simulink model "set_point"  (R2023b)
settings: Solver=VariableStepAuto  StartTime=0.0  StopTime=10.0  RelTol=1e-3
values from neighbouring files (symbols this model uses):
  r = 120.0    (= 120)    [controlador_foc_simulink.m]    (also in parametros_planta.m; params_subsistema_mecanico.m; sistema_completo_en_codigo.m)
settings Model: Creator=Pc  LastModifiedBy=Pc

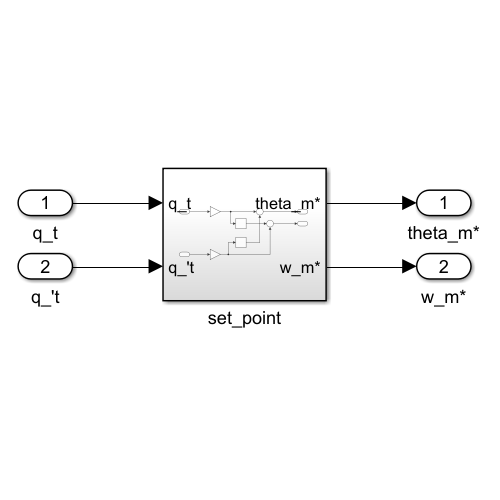
[thumbnail: Simulink's stored preview of the top-level diagram]
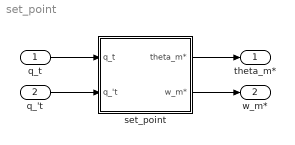
== system set_point ==
  q_t : Inport
  q_'t : Inport  Port=2
  set_point : Subsystem
  theta_m* : Outport
  w_m* : Outport  Port=2
  wires:
  q_t/1 -> set_point/1(q_t)
  q_'t/1 -> set_point/2(q_'t)
  set_point/1(theta_m*) -> theta_m*/1
  set_point/2(w_m*) -> w_m*/1

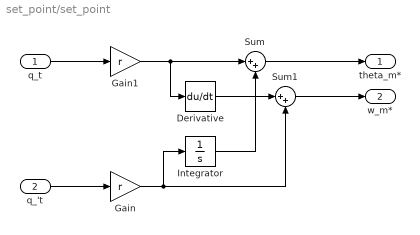
== system set_point/set_point ==
  q_t : Inport
  q_'t : Inport  Port=2
  Derivative : Derivative
  Gain : Gain  Gain=r
  Gain1 : Gain  Gain=r
  Integrator : Integrator
  Sum : Sum  Inputs=|++
  Sum1 : Sum  Inputs=|++
  theta_m* : Outport
  w_m* : Outport  Port=2
  wires:
  Gain1/1 -> Derivative/1, Sum/1
  Derivative/1 -> Sum1/1
  Gain/1 -> Integrator/1, Sum1/2
  Integrator/1 -> Sum/2
  Sum/1 -> theta_m*/1
  Sum1/1 -> w_m*/1
  q_'t/1 -> Gain/1
  q_t/1 -> Gain1/1
